simulink model "HW4_2b_least_squares_discrete_time"  (R2023b)
settings: Solver=VariableStepAuto  StartTime=0.0  StopTime=100  RelTol=1e-3
model workspace (MAT data in the model file):
  alpha = Simulink.Parameter
  alpha.Value = 1
  alpha.DataType = 'auto'
  alpha.Complexity = 'real'
  alpha.Dimensions = [1 1]
  b = Simulink.Parameter
  b.Value = 0.1
  b.DataType = 'auto'
  b.Complexity = 'real'
  b.Dimensions = [1 1]
  beta = Simulink.Parameter
  beta.Value = 1
  beta.DataType = 'auto'
  beta.Complexity = 'real'
  beta.Dimensions = [1 1]
  k = Simulink.Parameter
  k.Value = 5
  k.DataType = 'auto'
  k.Complexity = 'real'
  k.Dimensions = [1 1]
  m = Simulink.Parameter
  m.Value = 20
  m.DataType = 'auto'
  m.Complexity = 'real'
  m.Dimensions = [1 1]
  minv = Simulink.Parameter
  minv.Value = 0.05
  minv.DataType = 'auto'
  minv.Complexity = 'real'
  minv.Dimensions = [1 1]
undefined symbols (not defined in the file): DiscIntNeverNeededParam
libraries: matrix_library x3
settings Model: Creator=kaleb  LastModifiedBy=kaleb

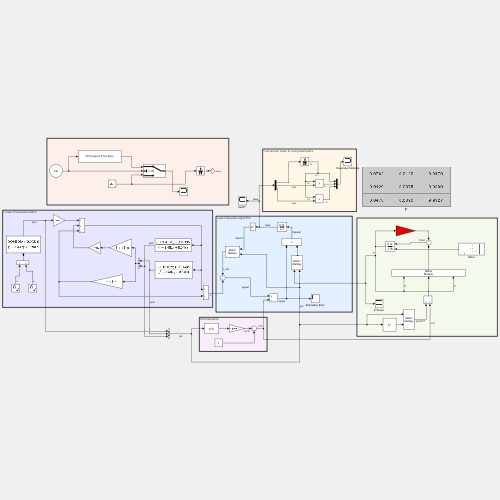
[thumbnail: Simulink's stored preview of the top-level diagram]
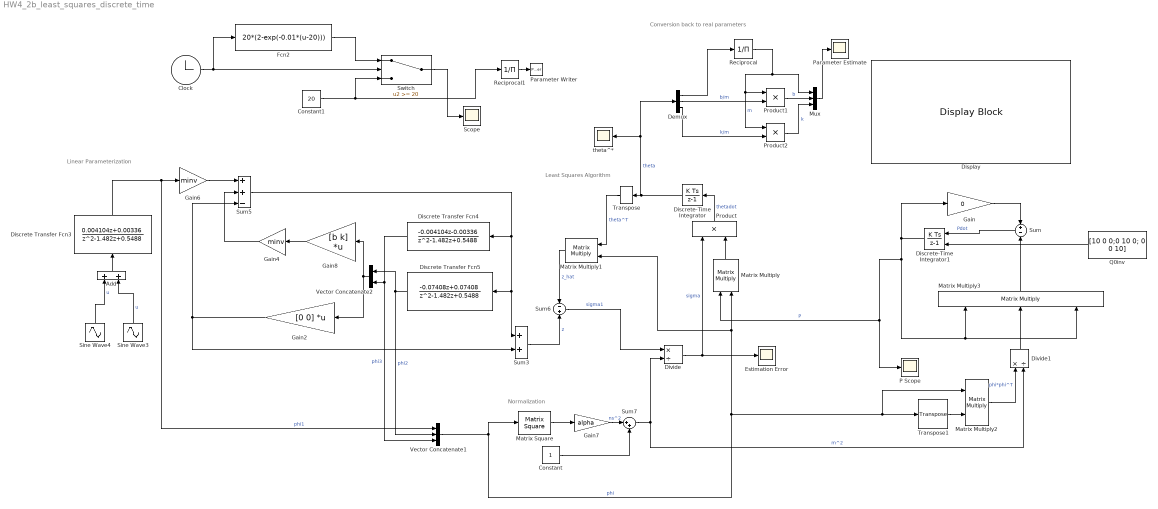
== system HW4_2b_least_squares_discrete_time ==
  note: Least Squares Algorithm
  note: Conversion back to real parameters
  note: Normalization
  note: Linear Parameterization
  Add : Sum
  Clock : Clock
  Constant : Constant
  Constant1 : Constant  Value=20
  Demux : Demux  Outputs=3
  Discrete Transfer Fcn3 : DiscreteTransferFcn  Numerator=[0.004104 0.00336]  Denominator=[1 -1.482 0.5488]
  Discrete Transfer Fcn4 : DiscreteTransferFcn  Numerator=[-0.004104 -0.00336]  Denominator=[1 -1.482 0.5488]
  Discrete Transfer Fcn5 : DiscreteTransferFcn  Numerator=[-0.07408 0.07408]  Denominator=[1 -1.482 0.5488]
  Discrete-Time Integrator : DiscreteIntegrator  InitialCondition=[0.1 0.1 0.1]  SampleTime=-1  ICPrevOutput=DiscIntNeverNeededParam  ICPrevScaledInput=DiscIntNeverNeededParam
  Discrete-Time Integrator1 : DiscreteIntegrator  InitialConditionSource=external  InitialCondition=[0.1 0.1 0.1]  SampleTime=-1  ICPrevOutput=DiscIntNeverNeededParam  ICPrevScaledInput=DiscIntNeverNeededParam
  Display : DisplayBlock  LabelPosition=Bottom  Transparency=1
  Divide : Product  Inputs=*/
  Divide1 : Product  Inputs=*/
  Estimation Error : Scope
  Fcn2 : Fcn  Expr=20*(2-exp(-0.01*(u-20)))
  Gain : Gain  Gain=0
  Gain2 : Gain  Gain=[0 0]  Multiplication=Matrix(K*u)
  Gain4 : Gain  Gain=minv
  Gain6 : Gain  Gain=minv
  Gain7 : Gain  Gain=alpha
  Gain8 : Gain  Gain=[b k]  Multiplication=Matrix(K*u)
  Matrix Square : matrix_library/Matrix Square  OutMin=[]  OutMax=[]
      settings: LibrarySourceBlock=|
      | simulink/Matrix
      | Operations/Matrix
      | Square
  Matrix Multiply : Product  Multiplication=Matrix(*)
  Matrix Multiply1 : Product  Multiplication=Matrix(*)
  Matrix Multiply2 : Product  Multiplication=Matrix(*)
  Matrix Multiply3 : Product  Inputs=3  Multiplication=Matrix(*)
  Mux : Mux  Inputs=3
  P Scope : Scope
  Parameter Estimate : Scope
  Parameter Writer : ParameterWriter  AccessWorkspaceVariable=on  WorkspaceVariableName=minv
  Product : Product
  Product1 : Product
  Product2 : Product
  Q0inv : Constant  Value=[10 0 0;0 10 0; 0 0 10]
  Reciprocal : Product  Inputs=/  OutMax=[10000]
  Reciprocal1 : Product  Inputs=/
  Scope : Scope
  Sine Wave3 : Sin  Amplitude=5  Frequency=0.5  SampleTime=0.1
  Sine Wave4 : Sin  Amplitude=2  Frequency=2  SampleTime=0.1
  Sum : Sum  Inputs=+-
  Sum3 : Sum
  Sum5 : Sum  Inputs=++-
  Sum6 : Sum  Inputs=-+
  Sum7 : Sum  Inputs=|++
  Switch : Switch  Threshold=20  ZeroCross=off  SaturateOnIntegerOverflow=off  InputSameDT=off
  Transpose : matrix_library/Transpose
  Transpose1 : matrix_library/Transpose
  Vector Concatenate1 : Concatenate  NumInputs=3
  Vector Concatenate2 : Concatenate
  theta^* : Scope
  wires:
  Matrix Multiply1/1 -> Sum6/1  "z_hat"
  Matrix Square/1 -> Gain7/1
  Constant/1 -> Sum7/2
  Sum7/1 -> Divide1/2, Divide/2  "m^2"
  Gain7/1 -> Sum7/1  "ns^2"
  Sum6/1 -> Divide/1  "sigma1"
  Product/1 -> Discrete-Time Integrator/1  "thetadot"
  Discrete-Time Integrator/1 -> Transpose/1, Demux/1, theta^*/1  "theta"
  Transpose/1 -> Matrix Multiply1/1  "theta^T"
  Divide/1 -> Estimation Error/1, Product/1  "sigma"
  Demux/2 -> Product1/2  "b/m"
  Demux/3 -> Product2/2  "k/m"
  Reciprocal/1 -> Product1/1, Product2/1, Mux/1  "m"
  Product1/1 -> Mux/2  "b"
  Product2/1 -> Mux/3  "k"
  Mux/1 -> Parameter Estimate/1
  Matrix Multiply/1 -> Product/2
  Demux/1 -> Reciprocal/1
  Discrete-Time Integrator1/1 -> Gain/1, Matrix Multiply/1, P Scope/1, Matrix Multiply3/3, Matrix Multiply3/1  "P"
  Gain/1 -> Sum/1
  Transpose1/1 -> Matrix Multiply2/2
  Matrix Multiply2/1 -> Divide1/1  "phi*phi^T"
  Matrix Multiply3/1 -> Sum/2
  Divide1/1 -> Matrix Multiply3/2
  Clock/1 -> Fcn2/1, Switch/2
  Constant1/1 -> Switch/3, Reciprocal1/1
  Fcn2/1 -> Switch/1
  Switch/1 -> Scope/1
  Reciprocal1/1 -> Parameter Writer/1
  Q0inv/1 -> Discrete-Time Integrator1/2
  Sum/1 -> Discrete-Time Integrator1/1  "Pdot"
  Sine Wave4/1 -> Add/1  "u"
  Sum3/1 -> Sum6/2  "z"
  Discrete Transfer Fcn5/1 -> Vector Concatenate1/2, Vector Concatenate2/1  "phi2"
  Gain4/1 -> Sum5/2
  Add/1 -> Discrete Transfer Fcn3/1
  Gain2/1 -> Sum5/3, Sum3/2
  Gain8/1 -> Gain4/1
  Discrete Transfer Fcn4/1 -> Vector Concatenate1/3, Vector Concatenate2/2  "phi3"
  Gain6/1 -> Sum5/1
  Vector Concatenate2/1 -> Gain8/1, Gain2/1
  Sine Wave3/1 -> Add/2  "u"
  Discrete Transfer Fcn3/1 -> Vector Concatenate1/1, Gain6/1  "phi1"
  Sum5/1 -> Discrete Transfer Fcn4/1, Sum3/1, Discrete Transfer Fcn5/1
  Vector Concatenate1/1 -> Matrix Multiply2/1, Transpose1/1, Matrix Multiply1/2, Matrix Multiply/2, Matrix Square/1  "phi"
